simulink model "noises"  (R2017a)
settings: Solver=VariableStepAuto  StartTime=0.0  StopTime=10.0  RelTol=1e-3
model workspace (MATLAB code in the model file):
  | N = 10;
  | simulation_step = 0.1;
settings Model: Creator=ignacio  LastModifiedBy=ignacio

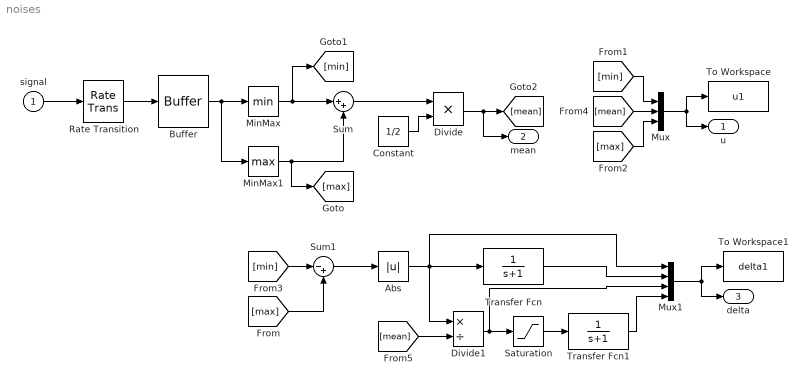
== system noises ==
  signal : Inport
  Abs : Abs
  Buffer : Buffer  N=N  V=N - 1  OutputFrames=off
  Constant : Constant  Value=1/2
  Divide : Product  SaturateOnIntegerOverflow=on  RndMeth=Zero
  Divide1 : Product  Inputs=*/  SaturateOnIntegerOverflow=on  RndMeth=Zero
  MinMax : MinMax
  MinMax1 : MinMax  Function=max
  Mux : Mux  Inputs=3
  Mux1 : Mux
  Rate Transition : RateTransition  OutPortSampleTime=simulation_step
  Saturation : Saturate  UpperLimit=800  LowerLimit=-800
  Sum : Sum  Inputs=|++
  Sum1 : Sum  Inputs=|-+
  To Workspace : ToWorkspace  VariableName=u1  SaveFormat=Timeseries  SampleTime=-1
  To Workspace1 : ToWorkspace  VariableName=delta1  SaveFormat=Timeseries  SampleTime=-1
  Transfer Fcn : TransferFcn  Denominator=[1 1]
  Transfer Fcn1 : TransferFcn  Denominator=[1 1]
  u : Outport
  mean : Outport  Port=2
  delta : Outport  Port=3
  wires:
  Divide/1 -> mean/1, [mean]
  [max] -> Sum1/2
  Sum/1 -> Divide/1
  Mux/1 -> u/1, To Workspace/1
  Sum1/1 -> Abs/1
  Rate Transition/1 -> Buffer/1
  [mean] -> Mux/2
  Constant/1 -> Divide/2
  Transfer Fcn/1 -> Mux1/2
  [mean] -> Divide1/2
  [max] -> Mux/3
  Transfer Fcn1/1 -> Mux1/4
  MinMax/1 -> [min], Sum/1
  MinMax1/1 -> Sum/2, [max]
  Buffer/1 -> MinMax1/1, MinMax/1
  Abs/1 -> Mux1/1, Divide1/1, Transfer Fcn/1
  Saturation/1 -> Transfer Fcn1/1
  Mux1/1 -> To Workspace1/1, delta/1
  Divide1/1 -> Saturation/1, Mux1/3
  [min] -> Sum1/1
  signal/1 -> Rate Transition/1
  [min] -> Mux/1
